simulink model "uav_6dof"  (R2020b)
settings: Solver=VariableStepAuto  StartTime=0.0  StopTime=20  RelTol=1e-3
libraries: simulink x1
settings Model: Creator=Christie  LastModifiedBy=Christie

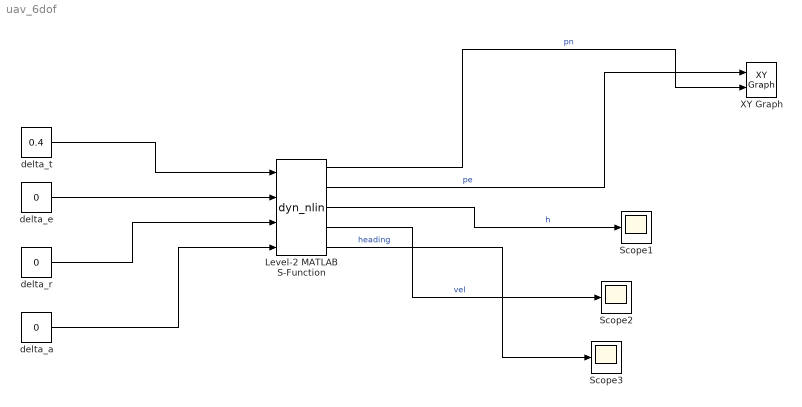
== system uav_6dof ==
  Level-2 MATLAB S-Function : M-S-Function  FunctionName=dyn_nlin
  Scope1 : Scope
  Scope2 : Scope
  Scope3 : Scope
  XY Graph : simulink/Sinks/XY Graph  xmin=0  xmax=inf  ymin=0  ymax=inf  st=-1
  delta_a : Constant  Value=0
  delta_e : Constant  Value=0
  delta_r : Constant  Value=0
  delta_t : Constant  Value=0.4
  wires:
  delta_t/1 -> Level-2 MATLAB S-Function/1
  delta_e/1 -> Level-2 MATLAB S-Function/2
  Level-2 MATLAB S-Function/1 -> XY Graph/2  "pn"
  Level-2 MATLAB S-Function/2 -> XY Graph/1  "pe"
  delta_r/1 -> Level-2 MATLAB S-Function/3
  delta_a/1 -> Level-2 MATLAB S-Function/4
  Level-2 MATLAB S-Function/3 -> Scope1/1  "h"
  Level-2 MATLAB S-Function/4 -> Scope2/1  "vel"
  Level-2 MATLAB S-Function/5 -> Scope3/1  "heading"
